simulink model "lap2part1slx"  (R2021a)
settings: Solver=VariableStepAuto  StartTime=0.0  StopTime=10.0  RelTol=1e-3
settings Model: Creator=USER59  LastModifiedBy=USER59

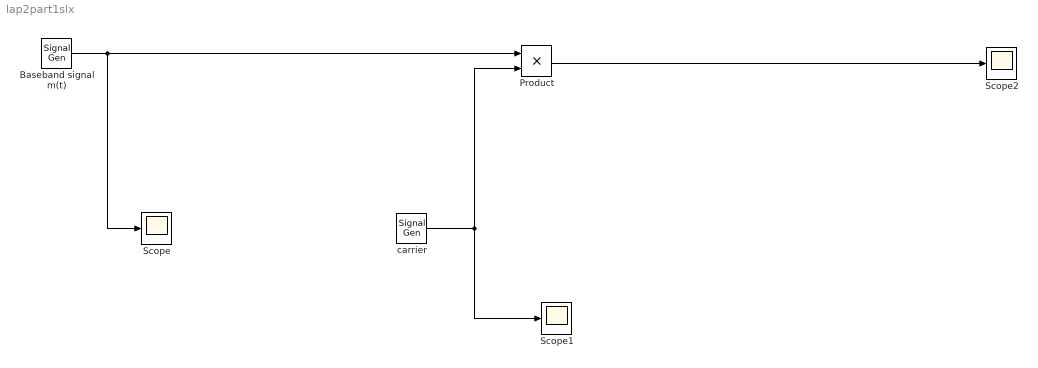
== system lap2part1slx ==
  Baseband signal m(t) : SignalGenerator  Frequency=1000  Units=rad/sec
  Product : Product
  Scope : Scope
  Scope1 : Scope
  Scope2 : Scope
  carrier : SignalGenerator  Amplitude=5  Frequency=50000  Units=rad/sec
  wires:
  Baseband signal m(t)/1 -> Scope/1, Product/1
  carrier/1 -> Scope1/1, Product/2
  Product/1 -> Scope2/1
